simulink model "lab_elev_travel"  (Simulink 8.6)
settings: Solver=ode1  StartTime=0.0  StopTime=inf  FixedStep=0.002  RelTol=1e-3
values from neighbouring files (symbols this model uses):
  C = [1,0,0,0,0,0;0,0,1,0,0,0]    [lab_init.m]    (also in o_lqi.m = [1,0,0,0,0; 0,0,0,0,1])
  CMD_ELEV_POS_LIMIT_LOWER = elev_0*180/pi    (= -27.5)    [setup_lab_heli_3d.m]    (also in setup_lab_heli_3d_simple.m; setup_lab_heli_3d_various_controler.m; setup_lab_heli_3d_various_controler_with_Kalman_Filter.m)
  CMD_ELEV_POS_LIMIT_UPPER = -CMD_ELEV_POS_LIMIT_LOWER    (= 27.5)    [setup_lab_heli_3d.m]    (also in setup_lab_heli_3d_simple.m; setup_lab_heli_3d_various_controler.m; setup_lab_heli_3d_various_controler_with_Kalman_Filter.m)
  CMD_RATE_LIMIT = 45.0 * pi / 180    (= 0.785398163397)    [setup_lab_heli_3d.m]    (also in setup_lab_heli_3d_simple.m; setup_lab_heli_3d_various_controler.m; setup_lab_heli_3d_various_controler_with_Kalman_Filter.m)
  elev_0 = -27.5*pi/180    (= -0.479965544298)    [setup_lab_heli_3d.m]    (also in setup_lab_heli_3d_simple.m; setup_lab_heli_3d_various_controler.m; setup_lab_heli_3d_various_controler_with_Kalman_Filter.m)
  K = lqr(A,B,Q_x,Q_u)    [lab_init.m]    (also in setup_lab_heli_3d.m = zeros(2,6); setup_lab_heli_3d_various_controler.m = lqr( Ai, Bi, Q, R ); setup_lab_heli_3d_various_controler_with_Kalman_Filter.m = lqr( Ai, Bi, Q, R ))
  K_AMP = 3    [setup_lab_heli_3d.m]    (also in setup_lab_heli_3d_simple.m; setup_lab_heli_3d_various_controler.m; setup_lab_heli_3d_various_controler_with_Kalman_Filter.m)
  K_I = zeros(2)    [lab_init.m]
  K_JOYSTICK_X = 40.0    (= 40)    [setup_lab_heli_3d.m]    (also in setup_lab_heli_3d_simple.m; setup_lab_heli_3d_various_controler.m; setup_lab_heli_3d_various_controler_with_Kalman_Filter.m)
  K_JOYSTICK_Y = 45.0    (= 45)    [setup_lab_heli_3d.m]    (also in setup_lab_heli_3d_simple.m; setup_lab_heli_3d_various_controler.m; setup_lab_heli_3d_various_controler_with_Kalman_Filter.m)
  K_r = inv(C*inv(-A+B*K)*B)    [lab_init.m]
  SAT_INT_ERR_TRAVEL = 7.5    [setup_lab_heli_3d.m]    (also in setup_lab_heli_3d_simple.m; setup_lab_heli_3d_various_controler.m; setup_lab_heli_3d_various_controler_with_Kalman_Filter.m)
  V_K = 0    [lab_init.m]
  VMAX_AMP = 24    [setup_lab_heli_3d.m]    (also in setup_lab_heli_3d_simple.m; setup_lab_heli_3d_various_controler.m; setup_lab_heli_3d_various_controler_with_Kalman_Filter.m)
  VMAX_DAC = 10    [setup_lab_heli_3d.m]    (also in setup_lab_heli_3d_simple.m; setup_lab_heli_3d_various_controler.m; setup_lab_heli_3d_various_controler_with_Kalman_Filter.m)
  wcf = 2 * pi * 2.5    (= 15.7079632679)    [setup_ads_configuration.m]    (also in setup_lab_heli_3d.m = 125.663706144; setup_lab_heli_3d_simple.m = 125.663706144; setup_lab_heli_3d_various_controler.m = 125.663706144; setup_lab_heli_3d_various_controler_with_Kalman_Filter.m = 125.663706144)
  zetaf = 0.9    [setup_lab_heli_3d.m]    (also in setup_lab_heli_3d_simple.m; setup_lab_heli_3d_various_controler.m; setup_lab_heli_3d_various_controler_with_Kalman_Filter.m)
undefined symbols (not defined in the file or in its folder): CMD_TRAVEL_POS_LIMIT_LOWER, CMD_TRAVEL_POS_LIMIT_UPPER, HIL, K_EC_E, K_EC_P, K_EC_T, qc_get_step_size
libraries: quarc_library x5, simulink_extras x4, simulink x2
settings Model: Creator=MLevis  LastModifiedBy=giugio  SimulationMode=external  ExtModeTrigDuration=10000
settings SolverCC: PositivePriorityOrder=on
settings OptimizationCC: InitFltsAndDblsToZero=on
settings DebuggingCC: SaveWithParameterizedLinksMsg=none  FcnCallInpInsideContextMsg=UseLocalSettings  StrictBusMsg=Warning
settings RTWCC: SystemTargetFile=quarc_win64.tlc  TemplateMakefile=quarc_default_tmf  Description=QUARC Win64 Target
settings STFCustomTargetCC: TargetPreCompLibLocation=C:\PROGRA~3\QUARC\lib\2015b\win64\release  GeneratePreprocessorConditionals=Disable all  CPPClassGenCompliant=on  SystemTargetFile=quarc_win64.tlc
settings GRTTargetCC: TargetPreCompLibLocation=C:\PROGRA~3\QUARC\lib\2015b\win64\release  ParMdlRefBuildCompliant=off  CompOptLevelCompliant=off  ConcurrentExecutionCompliant=off  MatFileLogging=off  UseToolchainInfoCompliant=off  ExtMode=on  ExtModeMexFile=quarc_comm

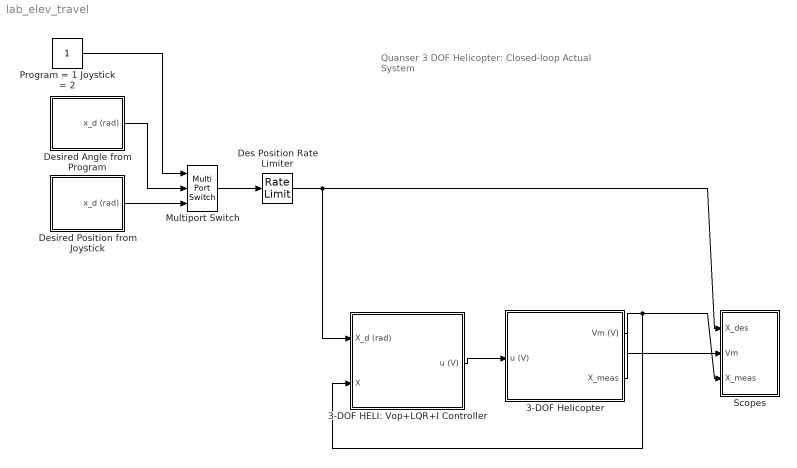
== system lab_elev_travel ==
  note: Quanser 3 DOF Helicopter:
      | Closed-loop Actual System
  3-DOF HELI: Vop+LQR+I Controller : Subsystem
  3-DOF Helicopter : Subsystem
  Des Position Rate Limiter : RateLimiter  RisingSlewLimit=CMD_RATE_LIMIT  FallingSlewLimit=-CMD_RATE_LIMIT  SampleTimeMode=inherited
  Desired Angle from Program : Subsystem
  Desired Position from Joystick : Subsystem
  Multiport Switch : MultiPortSwitch  Inputs=2
  Program = 1 Joystick = 2 : Constant
  Scopes : Subsystem
  wires:
  3-DOF Helicopter/1(Vm (V)) -> Scopes/2(Vm)
  3-DOF Helicopter/2(X_meas) -> Scopes/3(X_meas), 3-DOF HELI: Vop+LQR+I Controller/2(X)
  Des Position Rate Limiter/1 -> Scopes/1(X_des), 3-DOF HELI: Vop+LQR+I Controller/1(X_d (rad))
  Program = 1 Joystick = 2/1 -> Multiport Switch/1
  Desired Angle from Program/1(x_d (rad)) -> Multiport Switch/2
  Desired Position from Joystick/1(x_d (rad)) -> Multiport Switch/3
  Multiport Switch/1 -> Des Position Rate Limiter/1
  3-DOF HELI: Vop+LQR+I Controller/1(u (V)) -> 3-DOF Helicopter/1(u (V))

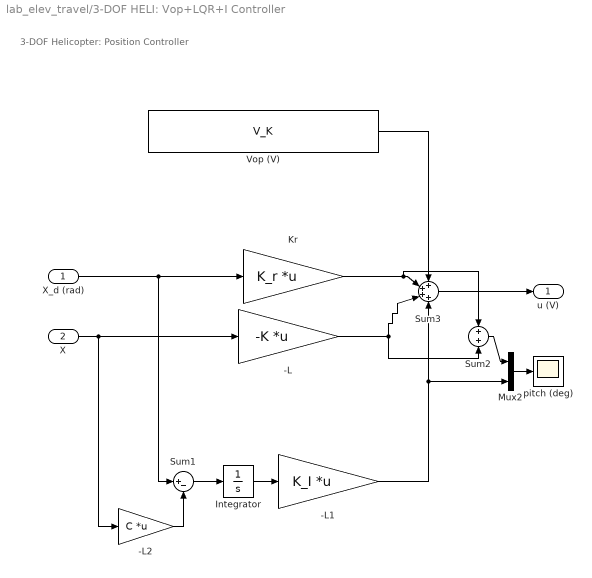
== system lab_elev_travel/3-DOF HELI: Vop+LQR+I Controller ==
  note: 3-DOF Helicopter: Position Controller
  X_d (rad) : Inport
  X : Inport  Port=2
  -L : Gain  Gain=-K  Multiplication=Matrix(K*u)
  -L1 : Gain  Gain=K_I  Multiplication=Matrix(K*u)
  -L2 : Gain  Gain=C  Multiplication=Matrix(K*u)
  Integrator : Integrator  LimitOutput=on  UpperSaturationLimit=SAT_INT_ERR_TRAVEL  LowerSaturationLimit=-SAT_INT_ERR_TRAVEL
  Kr : Gain  Gain=K_r  Multiplication=Matrix(K*u)
  Mux2 : Mux  Inputs=2
  Sum1 : Sum  Inputs=|+-
  Sum2 : Sum
  Sum3 : Sum  Inputs=++++
  Vop (V) : Constant  Value=V_K
  pitch (deg) : Scope
  u (V) : Outport
  wires:
  X_d (rad)/1 -> Kr/1, Sum1/1
  X/1 -> -L/1, -L2/1
  Sum3/1 -> u (V)/1
  Vop (V)/1 -> Sum3/1
  Kr/1 -> Sum3/2, Sum2/1
  -L/1 -> Sum3/3, Sum2/2
  -L1/1 -> Sum3/4, Mux2/2
  Integrator/1 -> -L1/1
  Sum1/1 -> Integrator/1
  -L2/1 -> Sum1/2
  Sum2/1 -> Mux2/1
  Mux2/1 -> pitch (deg)/1

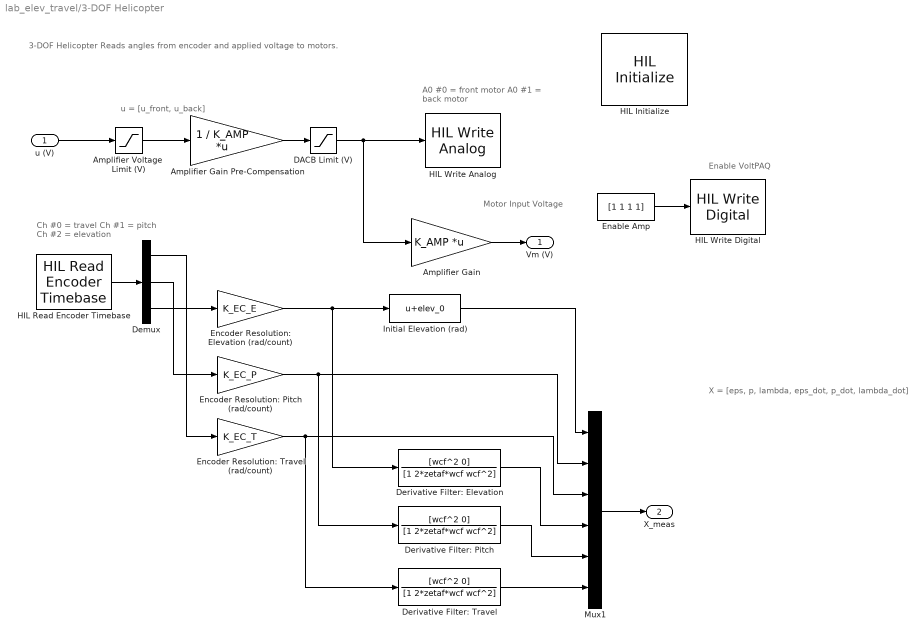
== system lab_elev_travel/3-DOF Helicopter ==
  note: A0 #0 = front motor
      | A0 #1 = back motor
  note: u = [u_front, u_back]
  note: Motor Input Voltage
  note: 3-DOF Helicopter
      | Reads angles from encoder and applied voltage to motors.
  note: Ch #0 = travel
      | Ch #1 = pitch
      | Ch #2 = elevation
  note: X = [eps, p, lambda, eps_dot, p_dot, lambda_dot]
  note: Enable VoltPAQ
  u (V) : Inport
  Amplifier Gain : Gain  Gain=K_AMP  Multiplication=Matrix(K*u)  SaturateOnIntegerOverflow=on  OutDataTypeStr=Inherit: Same as input  ParamDataTypeStr=Inherit: Same as input
  Amplifier Gain Pre-Compensation : Gain  Gain=1 / K_AMP  Multiplication=Matrix(K*u)  SaturateOnIntegerOverflow=on  OutDataTypeStr=Inherit: Same as input  ParamDataTypeStr=Inherit: Same as input
  Amplifier Voltage  Limit (V) : Saturate  UpperLimit=VMAX_AMP  LowerLimit=-VMAX_AMP
  DACB Limit (V) : Saturate  UpperLimit=VMAX_DAC  LowerLimit=-VMAX_DAC
  Demux : Demux  Outputs=3
  Derivative Filter: Elevation : TransferFcn  Numerator=[wcf^2 0]  Denominator=[1 2*zetaf*wcf wcf^2]
  Derivative Filter: Pitch : TransferFcn  Numerator=[wcf^2 0]  Denominator=[1 2*zetaf*wcf wcf^2]
  Derivative Filter: Travel : TransferFcn  Numerator=[wcf^2 0]  Denominator=[1 2*zetaf*wcf wcf^2]
  Enable Amp : Constant  Value=[1 1 1 1]
  Encoder Resolution: Elevation (rad/count) : Gain  Gain=K_EC_E
  Encoder Resolution: Pitch (rad/count) : Gain  Gain=K_EC_P
  Encoder Resolution: Travel (rad/count) : Gain  Gain=K_EC_T
  HIL Initialize : quarc_library/Data Acquisition/Generic/Configuration/HIL Initialize  object_name=HIL-1  board_type=q8_usb  board_number=0  board_options=update_rate=normal  exclusive=off  active=on  hardware_clocks=[0:2]  clock_modes=[]  initial_clock_frequencies=[]  set_clock_params_at_start=off  set_clock_params_at_switch_in=off  set_clock_frequencies_at_start=off  set_clock_frequencies_at_switch_in=off  analog_input_channels=[0:7]  analog_input_maximums=10  analog_input_minimums=-10  set_analog_input_params_at_start=on  set_analog_input_params_at_switch_in=off  analog_output_channels=[0:7]  analog_output_maximums=10  analog_output_minimums=-10  initial_analog_outputs=[0]  final_analog_outputs=[0]  watchdog_analog_outputs=0  set_analog_output_params_at_start=on  set_analog_output_params_at_switch_in=off  set_analog_outputs_at_start=on  set_analog_outputs_at_switch_in=off  set_analog_outputs_at_terminate=on  set_analog_outputs_at_switch_out=off  set_analog_outputs_on_watchdog=off  digital_input_channels=[4:7]  digital_output_channels=[0:3]  digital_output_configuration=[]  initial_digital_outputs=[0]  final_digital_outputs=[0]  watchdog_digital_outputs=[0]  set_digital_output_params_at_start=off  set_digital_output_params_at_switch_in=off  set_digital_outputs_at_start=on  set_digital_outputs_at_switch_in=off  set_digital_outputs_at_terminate=on  set_digital_outputs_at_switch_out=off  set_digital_outputs_on_watchdog=off  encoder_channels=[0:7]  quadrature=[4]  encoder_filter_frequency=[]  initial_encoder_counts=[0]  set_encoder_params_at_start=on  set_encoder_params_at_switch_in=off  set_encoder_counts_at_start=on  set_encoder_counts_at_switch_in=off  pwm_channels=[0:7]  pwm_modes=0  pwm_frequency=99.532799999999995e6/4095  pwm_configuration=[0]  pwm_alignment=[0]  pwm_polarity=[1]  pwm_leading_deadband=[0]  pwm_trailing_deadband=[0]  initial_pwm_outputs=[0]  final_pwm_outputs=[0]  watchdog_pwm_outputs=[0]  set_pwm_params_at_start=on  set_pwm_params_at_switch_in=off  set_pwm_outputs_at_start=on  set_pwm_outputs_at_switch_in=off  set_pwm_outputs_at_terminate=on  set_pwm_outputs_at_switch_out=off  set_pwm_outputs_on_watchdog=off  other_output_channels=[]  initial_other_outputs=[]  final_other_outputs=[]  watchdog_other_outputs=[]  set_other_outputs_at_start=off  set_other_outputs_at_switch_in=off  set_other_outputs_at_terminate=off  set_other_outputs_at_switch_out=off  set_other_outputs_on_watchdog=off
  HIL Read Encoder Timebase : quarc_library/Data Acquisition/Generic/Timebases/HIL Read Encoder Timebase  object_name=HIL-1  clock=0  channels=[0:2]  samples_in_buffer=max(ceil(1/qc_get_step_size), 1)  active=on  vector_output=on  data_type_mode=Inherit via back propagation  data_type=double
  HIL Write Analog : quarc_library/Data Acquisition/Generic/Immediate I//O/HIL Write Analog  object_name=HIL-1  channels=[0,1]  sample_time=-1  active=off  vector_input=on
  HIL Write Digital : quarc_library/Data Acquisition/Generic/Immediate I//O/HIL Write Digital  object_name=HIL-1  channels=[0:3]  sample_time=-1  active=off  vector_input=on
  Initial Elevation (rad) : Bias  Bias=elev_0
  Mux1 : Mux  Inputs=6
  Vm (V) : Outport
  X_meas : Outport  Port=2
  wires:
  HIL Read Encoder Timebase/1 -> Demux/1
  Mux1/1 -> X_meas/1
  Amplifier Gain Pre-Compensation/1 -> DACB Limit (V)/1
  Amplifier Voltage  Limit (V)/1 -> Amplifier Gain Pre-Compensation/1
  Amplifier Gain/1 -> Vm (V)/1
  u (V)/1 -> Amplifier Voltage  Limit (V)/1
  DACB Limit (V)/1 -> Amplifier Gain/1, HIL Write Analog/1
  Demux/3 -> Encoder Resolution: Elevation (rad/count)/1
  Demux/1 -> Encoder Resolution: Travel (rad/count)/1
  Demux/2 -> Encoder Resolution: Pitch (rad/count)/1
  Encoder Resolution: Elevation (rad/count)/1 -> Derivative Filter: Elevation/1, Initial Elevation (rad)/1
  Encoder Resolution: Pitch (rad/count)/1 -> Mux1/2, Derivative Filter: Pitch/1
  Encoder Resolution: Travel (rad/count)/1 -> Mux1/3, Derivative Filter: Travel/1
  Derivative Filter: Elevation/1 -> Mux1/4
  Derivative Filter: Pitch/1 -> Mux1/5
  Derivative Filter: Travel/1 -> Mux1/6
  Initial Elevation (rad)/1 -> Mux1/1
  Enable Amp/1 -> HIL Write Digital/1

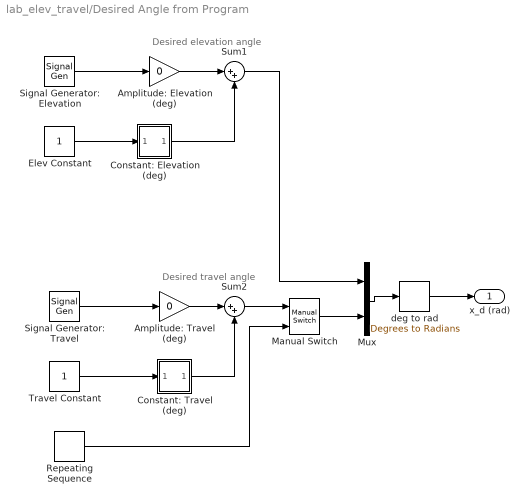
== system lab_elev_travel/Desired Angle from Program ==
  note: Desired travel angle
  note: Desired elevation angle
  Amplitude: Elevation (deg) : Gain  Gain=0
  Amplitude: Travel (deg) : Gain  Gain=0
  Constant: Elevation (deg) : Subsystem  LoadFcn=slideg Load  StartFcn=slideg StartFcn  StopFcn=slideg StopFcn  mask(Slider Gain){low=-27.5, gain=0, high=100}
      settings: CopyFcn=slideg Copy  DeleteFcn=slideg DeleteBlock  NameChangeFcn=slideg NameChange  OpenFcn=slideg Open  CloseFcn=slideg Close  ParentCloseFcn=slideg ParentClose
      mask Display: disp(gain)
  Constant: Travel (deg) : Subsystem  LoadFcn=slideg Load  StartFcn=slideg StartFcn  StopFcn=slideg StopFcn  mask(Slider Gain){low=-90, gain=0, high=90}
      settings: CopyFcn=slideg Copy  DeleteFcn=slideg DeleteBlock  NameChangeFcn=slideg NameChange  OpenFcn=slideg Open  CloseFcn=slideg Close  ParentCloseFcn=slideg ParentClose
      mask Display: disp(gain)
  Elev Constant : Constant
  Manual Switch : simulink/Signal Routing/Manual Switch  SystemSampleTime=-1  sw=1  action=0  varsize=off
  Mux : Mux  Inputs=2
  Repeating Sequence : simulink/Sources/Repeating Sequence  SystemSampleTime=-1  rep_seq_t="[0  15 16  30  45  46 60 ]"  rep_seq_y="[0 0 30 30  30 0 0 ]"
  Signal Generator: Elevation : SignalGenerator  WaveForm=square  Frequency=0.04
  Signal Generator: Travel : SignalGenerator  WaveForm=square  Frequency=0.05
  Sum1 : Sum  Inputs=|++
  Sum2 : Sum  Inputs=|++
  Travel Constant : Constant
  deg to rad : simulink_extras/Transformations/Degrees to Radians  SystemSampleTime=-1
  x_d (rad) : Outport
  wires:
  deg to rad/1 -> x_d (rad)/1
  Signal Generator: Travel/1 -> Amplitude: Travel (deg)/1
  Amplitude: Travel (deg)/1 -> Sum2/1
  Travel Constant/1 -> Constant: Travel (deg)/1(In1)
  Sum1/1 -> Mux/1
  Signal Generator: Elevation/1 -> Amplitude: Elevation (deg)/1
  Amplitude: Elevation (deg)/1 -> Sum1/1
  Mux/1 -> deg to rad/1
  Elev Constant/1 -> Constant: Elevation (deg)/1(In1)
  Constant: Elevation (deg)/1(Out1) -> Sum1/2
  Constant: Travel (deg)/1(Out1) -> Sum2/2
  Sum2/1 -> Manual Switch/1
  Manual Switch/1 -> Mux/2
  Repeating Sequence/1 -> Manual Switch/2

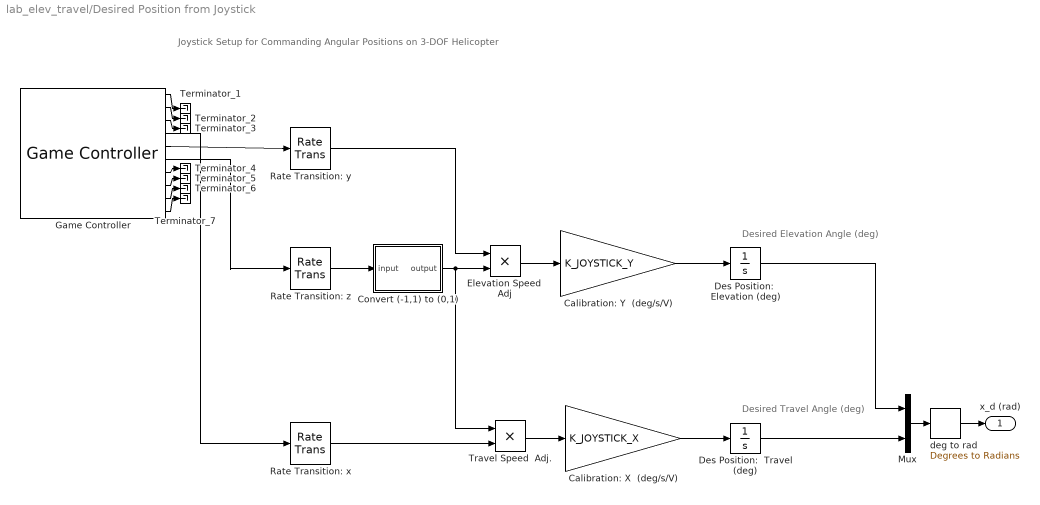
== system lab_elev_travel/Desired Position from Joystick ==
  note: Desired Elevation Angle (deg)
  note: Desired Travel Angle (deg)
  note: Joystick Setup for Commanding Angular Positions on 3-DOF Helicopter
  Calibration: X  (deg/s/V) : Gain  Gain=K_JOYSTICK_X
  Calibration: Y  (deg/s/V) : Gain  Gain=K_JOYSTICK_Y
  Convert (-1,1) to (0,1) : Subsystem
  Des Position:  Elevation (deg) : Integrator  InitialCondition=elev_0*180/pi  LimitOutput=on  UpperSaturationLimit=CMD_ELEV_POS_LIMIT_UPPER  LowerSaturationLimit=CMD_ELEV_POS_LIMIT_LOWER
  Des Position:  Travel (deg) : Integrator  UpperSaturationLimit=CMD_TRAVEL_POS_LIMIT_UPPER  LowerSaturationLimit=CMD_TRAVEL_POS_LIMIT_LOWER
  Elevation Speed  Adj : Product  RndMeth=Zero
  Game Controller : quarc_library/Devices/Peripherals/Target/Game Controller  controller=1  buffer_size=12  deadzone=[]  saturation=[]  sample_time=max(qc_get_step_size, 0.01)  auto_center=off  enabled=on
  Mux : Mux  Inputs=2
  Rate Transition: x : RateTransition
  Rate Transition: y : RateTransition
  Rate Transition: z : RateTransition
  Terminator_{1..7} (7 alike) : Terminator
  Travel Speed  Adj. : Product  RndMeth=Zero
  deg to rad : simulink_extras/Transformations/Degrees to Radians
  x_d (rad) : Outport
  wires:
  Des Position:  Elevation (deg)/1 -> Mux/1
  Des Position:  Travel (deg)/1 -> Mux/2
  Mux/1 -> deg to rad/1
  deg to rad/1 -> x_d (rad)/1
  Calibration: X  (deg/s/V)/1 -> Des Position:  Travel (deg)/1
  Travel Speed  Adj./1 -> Calibration: X  (deg/s/V)/1
  Elevation Speed  Adj/1 -> Calibration: Y  (deg/s/V)/1
  Calibration: Y  (deg/s/V)/1 -> Des Position:  Elevation (deg)/1
  Convert (-1,1) to (0,1)/1(output) -> Travel Speed  Adj./1, Elevation Speed  Adj/2
  Rate Transition: z/1 -> Convert (-1,1) to (0,1)/1(input)
  Rate Transition: y/1 -> Elevation Speed  Adj/1
  Rate Transition: x/1 -> Travel Speed  Adj./2
  Game Controller/5 -> Rate Transition: y/1
  Game Controller/6 -> Rate Transition: z/1
  Game Controller/4 -> Rate Transition: x/1
  Game Controller/1 -> Terminator_1/1
  Game Controller/2 -> Terminator_2/1
  Game Controller/3 -> Terminator_3/1
  Game Controller/7 -> Terminator_4/1
  Game Controller/8 -> Terminator_5/1
  Game Controller/9 -> Terminator_6/1
  Game Controller/10 -> Terminator_7/1

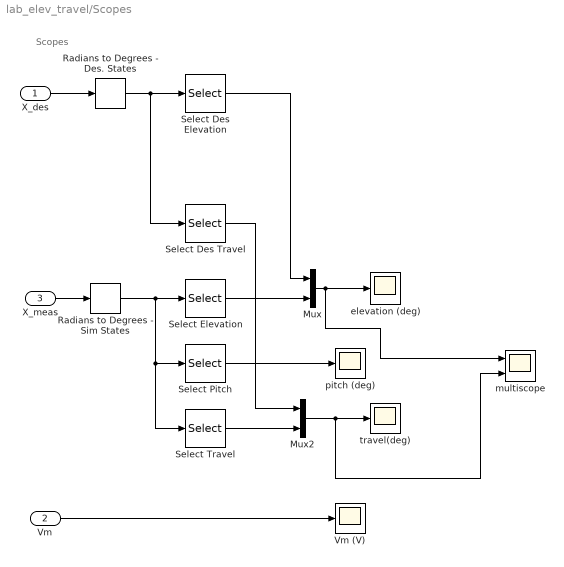
== system lab_elev_travel/Scopes ==
  note: Scopes
  X_des : Inport
  Vm : Inport  Port=2
  X_meas : Inport  Port=3
  Mux : Mux  Inputs=2
  Mux2 : Mux  Inputs=2
  Radians to Degrees - Des. States : simulink_extras/Transformations/Radians to Degrees
  Radians to Degrees - Sim States : simulink_extras/Transformations/Radians to Degrees
  Select Des Elevation : Selector  InputPortWidth=2  IndexOptions=Index vector (dialog)  Indices=1  OutputSizes=1
  Select Des Travel : Selector  InputPortWidth=2  IndexOptions=Index vector (dialog)  Indices=2  OutputSizes=1
  Select Elevation : Selector  InputPortWidth=6  IndexOptions=Index vector (dialog)  Indices=1  OutputSizes=1
  Select Pitch : Selector  InputPortWidth=6  IndexOptions=Index vector (dialog)  Indices=2  OutputSizes=1
  Select Travel : Selector  InputPortWidth=6  IndexOptions=Index vector (dialog)  Indices=3  OutputSizes=1
  Vm (V) : Scope
  elevation (deg) : Scope
  multiscope : Scope  NumInputPorts=2
  pitch (deg) : Scope
  travel(deg) : Scope
  wires:
  Select Des Travel/1 -> Mux2/1
  Select Des Elevation/1 -> Mux/1
  Radians to Degrees - Des. States/1 -> Select Des Elevation/1, Select Des Travel/1
  Select Travel/1 -> Mux2/2
  Select Pitch/1 -> pitch (deg)/1
  Select Elevation/1 -> Mux/2
  Mux2/1 -> travel(deg)/1, multiscope/2
  Radians to Degrees - Sim States/1 -> Select Travel/1, Select Pitch/1, Select Elevation/1
  Vm/1 -> Vm (V)/1
  Mux/1 -> elevation (deg)/1, multiscope/1
  X_meas/1 -> Radians to Degrees - Sim States/1
  X_des/1 -> Radians to Degrees - Des. States/1

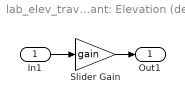
== system lab_elev_travel/Desired Angle from Program/Constant: Elevation (deg) ==
  In1 : Inport
  Slider Gain : Gain  Gain=gain  SaturateOnIntegerOverflow=on  OutDataTypeStr=Inherit: Same as input  ParamDataTypeStr=Inherit: Same as input
  Out1 : Outport
  wires:
  In1/1 -> Slider Gain/1
  Slider Gain/1 -> Out1/1

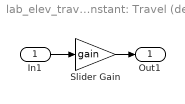
== system lab_elev_travel/Desired Angle from Program/Constant: Travel (deg) ==
  In1 : Inport
  Slider Gain : Gain  Gain=gain  SaturateOnIntegerOverflow=on  OutDataTypeStr=Inherit: Same as input  ParamDataTypeStr=Inherit: Same as input
  Out1 : Outport
  wires:
  In1/1 -> Slider Gain/1
  Slider Gain/1 -> Out1/1

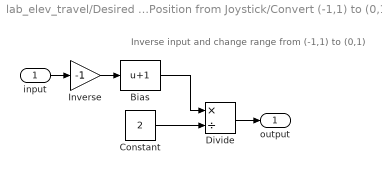
== system lab_elev_travel/Desired Position from Joystick/Convert (-1,1) to (0,1) ==
  note: Inverse input and change range from (-1,1) to (0,1)
  input : Inport
  Bias : Bias  Bias=1
  Constant : Constant  Value=2
  Divide : Product  Inputs=*/
  Inverse : Gain  Gain=-1
  output : Outport
  wires:
  Constant/1 -> Divide/2
  Bias/1 -> Divide/1
  input/1 -> Inverse/1
  Divide/1 -> output/1
  Inverse/1 -> Bias/1
